simulink library "gasLibrary"  (R2019a)
settings: Solver=VariableStepAuto  StartTime=0.0  StopTime=10.0  RelTol=1e-3
values from neighbouring files (symbols this model uses):
  loadControlFlag = "on"    [gas_v1.m]
undefined symbols (not defined in the file or in its folder): f
libraries: fl_lib x34, nesl_utility x12, instrumentlib x5
settings Model: Creator=dzimm  LastModifiedBy=brandt

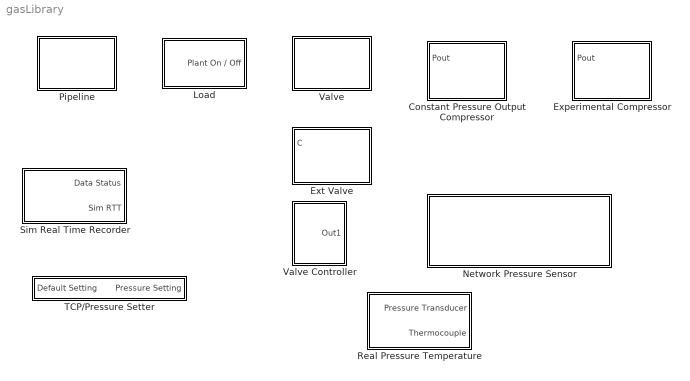
== system gasLibrary ==
  Constant Pressure Output Compressor : Subsystem  mask{xferNum=1, xferDen=[1800 1], delaySeconds=1, efficiency=0.3}
      mask prompts: xferNum "Plant Transfer Function Numerator (vector)"; xferDen "Plant Transfer Function Denominator (vector)"; delaySeconds "Response Delay (s)"; efficiency "Full Efficiency (-)"
  Experimental Compressor : Subsystem  AncestorBlock=gasLibrary/Constant Pressure Output Compressor  mask{xferNum=1, xferDen=[1800 1], delaySeconds=1, efficiency=0.3}
      mask prompts: xferNum "Plant Transfer Function Numerator (vector)"; xferDen "Plant Transfer Function Denominator (vector)"; delaySeconds "Response Delay (s)"; efficiency "Full Efficiency (-)"
  Ext Valve : Subsystem  AncestorBlock=gasLibrary/Valve  mask{valveRow=[], valveState="on"}
      mask prompts: valveRow "Valve Control (table row)"; valveState "Valve Simulation Control ('on' 'off' 'initial')"
      mask init:
      | if(isempty(valveRow)||isnumeric(valveRow))
      |     valveName="Valve";
      |     valveTime=[0 1e6]';
      |     valveSetting=[0 0]';
      |     D=20;           % size of the valve
      |     Dmax=D-1;       % maximum port opening
      |     textColor='red';
      | else
      |     valveName=valveRow.Name;
      |     t=valveRow.Time{1};
      |     g=valveRow.State{1};
      |     D=valveRow.PortDiameter;
      |     Dmax=valveRow.MaxValveDiameter;
      |     switch(lower(valveState))
      |         case "on"
      |             valveTime=t(:);
      |             valveSetting=g(:);
      |             textColor='green';
      |         case "off"
      |             valveTime=[0 1e6]';
      |             valveSetting=[1 1]';
      |             textColor='red';
      |         case "initial"
      |             valveTime=[0 1e6 ]';   % ramp gas on over one day
      |             valveSetting=[g(1)    g(1)]';     % gas ends at initial value
      |             textColor='blue';
      |         otherwise
      |             fprintf("Cannot initialize\n");
      |             textColor='green';
      |     end
      | end
      mask Display:
      | set_param(gcb,'Name',valveName);
      | color(textColor);
      | if(valveState=="off")
      |     vLabel="bypass";
      | else
      |     vLabel="active";
      | end
      | text(0.1,0.8,sprintf("%s (%1d in)",vLabel,D))
      | plot([0.2 0.9],[0.3 0.3]);
      | plot([0.2 0.2],[0.1 0.6]);
      | plot(valveTime/max(valveTime)*0.65+0.2,double(valveSetting)*0.4+0.15);
  Load : Subsystem  mask{loadRow=0, loadState=loadControlFlag}
      mask prompts: loadRow "Load Parameters (table row)"; loadState "Load Simulation Control ('on','off','initial')"
      mask init:
      | if(isempty(loadRow)||isnumeric(loadRow))
      |     loadName="Load";
      |     gasTime=[0 1e6]';
      |     gasLoad=[0 0]';
      |     textColor='red';
      |     pNominal=300;
      |     pCutoff=150;
      | else
      |     loadName=loadRow.Name;
      |     t=loadRow.Time{1};
      |     g=loadRow.Load{1};
      |     pNominal=loadRow.NominalPressure;
      |     pCutoff=loadRow.PressureCutoff;
      |     switch(lower(loadState))
      |         case "on"
      |             gasTime=t(:);
      |             gasLoad=g(:);
      |             textColor='green';
      |         case "off"
      |             gasTime=[0 1e6]';
      |             gasLoad=[0 0]';
      |             textColor='red';
      |         case "initial"
      |             gasTime=[0 24*3600 1e6 ]';   % ramp gas on over one day
      |             gasLoad=[0 g(1)    g(1)]';     % gas ends at initial value
      |             textColor='blue';
      |         otherwise
      |             fprintf("Cannot initialize\n");
      |             textColor='green';
      |     end
      | end
      mask Display:
      | tMax=max([gasTime(end)]);
      | set_param(gcb,'Name',loadName);
      | color(textColor);
      | text(0.1,0.8,sprintf("%s / %2.1f kg/s",loadState,max(gasLoad)))
      | plot([0.2 0.8],[0.1 0.1]);
      | plot([0.2 0.2],[0.1 0.6]);
      | plot(gasTime/tMax*0.6+0.2,gasLoad/max(gasLoad)*0.5+0.1);
  "Network Pressure Sensor " : Subsystem
  Pipeline : Subsystem  mask{pipeRow=[]}
      mask prompts: pipeRow "Pipeilne Configuration (table row)"
      mask init:
      | if(isempty(pipeRow))
      |     pipeName="Pipeline";
      |     D=24;
      |     L=50;
      |     Pstart=300;
      | else
      |     pipeName=pipeRow.Name;
      |     D=pipeRow.DiameterInch;
      |     L=pipeRow.LengthMiles;
      |     Pstart=pipeRow.StartPressurePSI;
      | end
      mask Display:
      | fprintf('%1d"\n%1d miles\n%1d psi',D,L,Pstart)
      | set_param(gcb,'Name',pipeName)
  Real Pressure Temperature : Subsystem  AncestorBlock=gasLibrary/Physical to Real Pressure Temperature
  Sim Real Time Recorder : Subsystem
  TCP/Pressure Setter : Subsystem
  Valve : Subsystem  mask{valveRow=[], valveState="on"}
      mask prompts: valveRow "Valve Control (table row)"; valveState "Valve Simulation Control ('on' 'off' 'initial')"
      mask init: same as gasLibrary/Ext Valve
      mask Display:
      | set_param(gcb,'Name',valveName);
      | color(textColor);
      | if(valveState=="off")
      |     vLabel="bypass";
      | else
      |     vLabel="active";
      | end
      | text(0.1,0.8,sprintf("%s (%1d in)",vLabel,D))
      | plot([0.2 0.9],[0.3 0.3]);
      | plot([0.2 0.2],[0.1 0.6]);
      | plot(valveTime/max(valveTime)*0.65+0.2,double(valveSetting)*0.4+0.15);
  Valve Controller : Subsystem

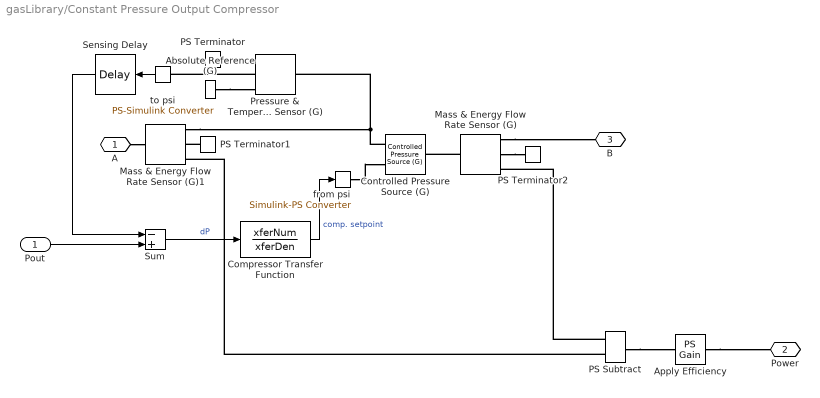
== system gasLibrary/Constant Pressure Output Compressor ==
  Pout : Inport
  Absolute Reference (G) : fl_lib/Gas/Elements/Absolute Reference (G)
      settings: SourceProductName=Simscape  SourceProductBaseCode=SS
  Apply Efficiency : fl_lib/Physical Signals/Functions/PS Gain  gain=1/efficiency
  Compressor Transfer Function : TransferFcn  Numerator=xferNum  Denominator=xferDen
  Controlled Pressure Source (G) : fl_lib/Gas/Sources/Controlled Pressure Source (G)  power_spec=1  area_A=24^2*pi/4 in^2  area_B=24^2*pi/4 in^2  mdot_A_specify=off  mdot_A_priority=None  mdot_A=1e-6 kg/s  mdot_A_nominal_specify=off  mdot_A_nominal_unit=kg/s  mdot_A_nominal_value=1
      settings: SourceProductName=Simscape  SourceProductBaseCode=SS
  Mass & Energy Flow Rate Sensor (G) : fl_lib/Gas/Sensors/Mass & Energy Flow Rate Sensor (G)
      settings: SourceProductName=Simscape  SourceProductBaseCode=SS
  Mass & Energy Flow Rate Sensor (G)1 : fl_lib/Gas/Sensors/Mass & Energy Flow Rate Sensor (G)
      settings: SourceProductName=Simscape  SourceProductBaseCode=SS
  PS Subtract : fl_lib/Physical Signals/Functions/PS Subtract
      settings: SourceProductName=Simscape
  PS Terminator : fl_lib/Physical Signals/Sinks/PS Terminator
      settings: SourceProductName=Simscape
  PS Terminator1 : fl_lib/Physical Signals/Sinks/PS Terminator
      settings: SourceProductName=Simscape
  PS Terminator2 : fl_lib/Physical Signals/Sinks/PS Terminator
      settings: SourceProductName=Simscape
  Pressure & Temperature Sensor (G) : fl_lib/Gas/Sensors/Pressure & Temperature Sensor (G)
      settings: SourceProductName=Simscape  SourceProductBaseCode=SS
  Sensing Delay : TransportDelay  DelayTime=delaySeconds  TransDelayFeedthrough=on
  Sum : Sum  Inputs=-+
  from psi : nesl_utility/Simulink-PS Converter  PhysicalDomain=network_engine_domain  SubClassName=ps_input  LeftPortType=input  RightPortType=output  PseudoPeriodic=off  Frequencies=[]  NoiseDistribution=none  NoiseParameters=[]  Unit=psi  AffineConversion=off  FilteringAndDerivatives=provide  SimscapeFilterOrder=1  InputFilterTimeConstant=0.001  UdotUserProvided=0
  to psi : nesl_utility/PS-Simulink Converter  PhysicalDomain=network_engine_domain  SubClassName=ps_output  LeftPortType=input  RightPortType=output  PseudoPeriodic=off  Frequencies=[]  Unit=psi  AffineConversion=off
  A : PMIOPort  Side=Left
  Power : PMIOPort  Port=2  Side=Right
  B : PMIOPort  Port=3  Side=Right
  wires:
  Pout/1 -> Sum/2
  Sum/1 -> Compressor Transfer Function/1  "dP"
  Compressor Transfer Function/1 -> from psi/1  "comp. setpoint"
  Sensing Delay/1 -> Sum/1
  to psi/1 -> Sensing Delay/1
  connections:
  Absolute Reference (G)/LConn1 -- Pressure & Temperature Sensor (G)/RConn1
  Pressure & Temperature Sensor (G)/RConn2 -- to psi/LConn1
  from psi/RConn1 -- Controlled Pressure Source (G)/LConn2
  PS Terminator/LConn1 -- Pressure & Temperature Sensor (G)/RConn3
  Controlled Pressure Source (G)/LConn1 -- Mass & Energy Flow Rate Sensor (G)1/RConn1 -- Pressure & Temperature Sensor (G)/LConn1
  Mass & Energy Flow Rate Sensor (G)/LConn1 -- Controlled Pressure Source (G)/RConn1
  Mass & Energy Flow Rate Sensor (G)/RConn1 -- B/RConn1
  A/RConn1 -- Mass & Energy Flow Rate Sensor (G)1/LConn1
  PS Terminator1/LConn1 -- Mass & Energy Flow Rate Sensor (G)1/RConn2
  Mass & Energy Flow Rate Sensor (G)/RConn2 -- PS Terminator2/LConn1
  PS Subtract/LConn1 -- Mass & Energy Flow Rate Sensor (G)/RConn3
  PS Subtract/LConn2 -- Mass & Energy Flow Rate Sensor (G)1/RConn3
  PS Subtract/RConn1 -- Apply Efficiency/LConn1
  Apply Efficiency/RConn1 -- Power/RConn1

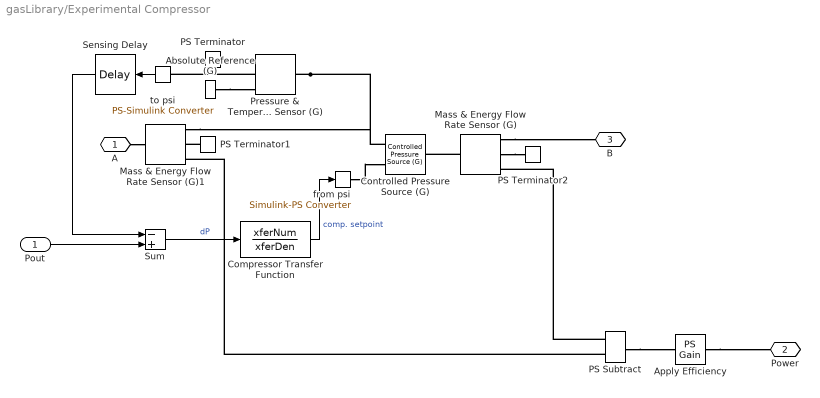
== system gasLibrary/Experimental Compressor ==
  Pout : Inport
  Absolute Reference (G) : fl_lib/Gas/Elements/Absolute Reference (G)
      settings: SourceProductName=Simscape  SourceProductBaseCode=SS
  Apply Efficiency : fl_lib/Physical Signals/Functions/PS Gain  gain=1/efficiency
  Compressor Transfer Function : TransferFcn  Numerator=xferNum  Denominator=xferDen
  Controlled Pressure Source (G) : fl_lib/Gas/Sources/Controlled Pressure Source (G)  power_spec=1  area_A=24^2*pi/4 in^2  area_B=24^2*pi/4 in^2  mdot_A_specify=off  mdot_A_priority=None  mdot_A=1e-6 kg/s  mdot_A_nominal_specify=off  mdot_A_nominal_unit=kg/s  mdot_A_nominal_value=1
      settings: SourceProductName=Simscape  SourceProductBaseCode=SS
  Mass & Energy Flow Rate Sensor (G) : fl_lib/Gas/Sensors/Mass & Energy Flow Rate Sensor (G)
      settings: SourceProductName=Simscape  SourceProductBaseCode=SS
  Mass & Energy Flow Rate Sensor (G)1 : fl_lib/Gas/Sensors/Mass & Energy Flow Rate Sensor (G)
      settings: SourceProductName=Simscape  SourceProductBaseCode=SS
  PS Subtract : fl_lib/Physical Signals/Functions/PS Subtract
      settings: SourceProductName=Simscape
  PS Terminator : fl_lib/Physical Signals/Sinks/PS Terminator
      settings: SourceProductName=Simscape
  PS Terminator1 : fl_lib/Physical Signals/Sinks/PS Terminator
      settings: SourceProductName=Simscape
  PS Terminator2 : fl_lib/Physical Signals/Sinks/PS Terminator
      settings: SourceProductName=Simscape
  Pressure & Temperature Sensor (G) : fl_lib/Gas/Sensors/Pressure & Temperature Sensor (G)
      settings: SourceProductName=Simscape  SourceProductBaseCode=SS
  Sensing Delay : TransportDelay  DelayTime=delaySeconds  TransDelayFeedthrough=on
  Sum : Sum  Inputs=-+
  from psi : nesl_utility/Simulink-PS Converter  PhysicalDomain=network_engine_domain  SubClassName=ps_input  LeftPortType=input  RightPortType=output  PseudoPeriodic=off  Frequencies=[]  NoiseDistribution=none  NoiseParameters=[]  Unit=psi  AffineConversion=off  FilteringAndDerivatives=provide  SimscapeFilterOrder=1  InputFilterTimeConstant=0.001  UdotUserProvided=0
  to psi : nesl_utility/PS-Simulink Converter  PhysicalDomain=network_engine_domain  SubClassName=ps_output  LeftPortType=input  RightPortType=output  PseudoPeriodic=off  Frequencies=[]  Unit=psi  AffineConversion=off
  A : PMIOPort  Side=Left
  Power : PMIOPort  Port=2  Side=Right
  B : PMIOPort  Port=3  Side=Right
  wires:
  to psi/1 -> Sensing Delay/1
  Sensing Delay/1 -> Sum/1
  Compressor Transfer Function/1 -> from psi/1  "comp. setpoint"
  Sum/1 -> Compressor Transfer Function/1  "dP"
  Pout/1 -> Sum/2
  connections:
  Apply Efficiency/RConn1 -- Power/RConn1
  PS Subtract/RConn1 -- Apply Efficiency/LConn1
  PS Subtract/LConn2 -- Mass & Energy Flow Rate Sensor (G)1/RConn3
  PS Subtract/LConn1 -- Mass & Energy Flow Rate Sensor (G)/RConn3
  Mass & Energy Flow Rate Sensor (G)/RConn2 -- PS Terminator2/LConn1
  PS Terminator1/LConn1 -- Mass & Energy Flow Rate Sensor (G)1/RConn2
  A/RConn1 -- Mass & Energy Flow Rate Sensor (G)1/LConn1
  Mass & Energy Flow Rate Sensor (G)/RConn1 -- B/RConn1
  Mass & Energy Flow Rate Sensor (G)/LConn1 -- Controlled Pressure Source (G)/RConn1
  Pressure & Temperature Sensor (G)/LConn1 -- Mass & Energy Flow Rate Sensor (G)1/RConn1 -- Controlled Pressure Source (G)/LConn1
  PS Terminator/LConn1 -- Pressure & Temperature Sensor (G)/RConn3
  from psi/RConn1 -- Controlled Pressure Source (G)/LConn2
  Pressure & Temperature Sensor (G)/RConn2 -- to psi/LConn1
  Absolute Reference (G)/LConn1 -- Pressure & Temperature Sensor (G)/RConn1

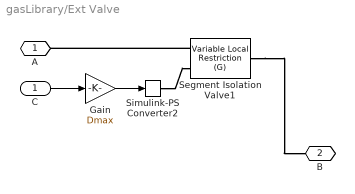
== system gasLibrary/Ext Valve ==
  C : Inport
  Gain : Gain  Gain=Dmax
  Segment Isolation Valve1 : fl_lib/Gas/Elements/Variable Local Restriction (G)  min_area=1e-4 in^2  max_area=pi*(Dmax-1)^2/4 in^2  area=pi*D^2/4 in^2  Cd=0.64  B_lam=0.999  mdot_A_specify=off  mdot_A_priority=None  mdot_A=1e-6 kg/s  mdot_A_nominal_specify=off  mdot_A_nominal_unit=kg/s  mdot_A_nominal_value=1
      settings: SourceProductName=Simscape  SourceProductBaseCode=SS
  Simulink-PS Converter2 : nesl_utility/Simulink-PS Converter  PhysicalDomain=network_engine_domain  SubClassName=ps_input  LeftPortType=input  RightPortType=output  PseudoPeriodic=off  Frequencies=[]  NoiseDistribution=none  NoiseParameters=[]  Unit=in^2  AffineConversion=off  FilteringAndDerivatives=provide  SimscapeFilterOrder=1  InputFilterTimeConstant=0.001  UdotUserProvided=0
  A : PMIOPort  Side=Left
  B : PMIOPort  Port=2  Side=Right
  wires:
  C/1 -> Gain/1
  Gain/1 -> Simulink-PS Converter2/1
  connections:
  Segment Isolation Valve1/RConn1 -- B/RConn1
  Segment Isolation Valve1/LConn1 -- A/RConn1
  Simulink-PS Converter2/RConn1 -- Segment Isolation Valve1/LConn2

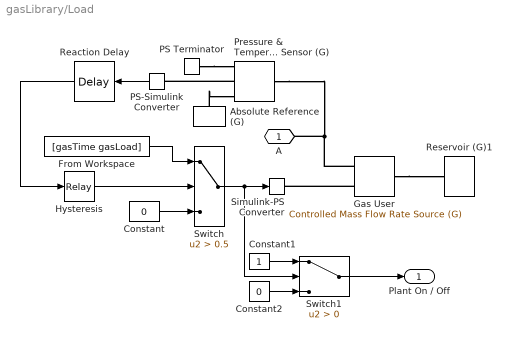
== system gasLibrary/Load ==
  Absolute Reference (G) : fl_lib/Gas/Elements/Absolute Reference (G)
      settings: SourceProductName=Simscape  SourceProductBaseCode=SS
  Constant : Constant  Value=0
  Constant1 : Constant
  Constant2 : Constant  Value=0
  From Workspace : FromWorkspace  VariableName=[gasTime gasLoad]  SampleTime=0  OutputAfterFinalValue=Holding final value
  Gas User : fl_lib/Gas/Sources/Controlled Mass Flow Rate Source (G)  power_spec=1  area_A=24^2*pi/4 in^2  area_B=20^2*pi/4 in^2  mdot_A_specify=on  mdot_A_priority=None  mdot_A=20 kg/s  mdot_A_nominal_specify=off  mdot_A_nominal_unit=kg/s  mdot_A_nominal_value=1
      settings: SourceProductName=Simscape  SourceProductBaseCode=SS
  Hysteresis : Relay  OnSwitchValue=pCutoff*1.05  OffSwitchValue=pCutoff
  PS Terminator : fl_lib/Physical Signals/Sinks/PS Terminator
      settings: SourceProductName=Simscape
  PS-Simulink Converter : nesl_utility/PS-Simulink Converter  PhysicalDomain=network_engine_domain  SubClassName=ps_output  LeftPortType=input  RightPortType=output  PseudoPeriodic=off  Frequencies=[]  Unit=psi  AffineConversion=off
  Pressure & Temperature Sensor (G) : fl_lib/Gas/Sensors/Pressure & Temperature Sensor (G)
      settings: SourceProductName=Simscape  SourceProductBaseCode=SS
  Reaction Delay : TransportDelay  DelayTime=60  InitialOutput=pNominal
  Reservoir (G)1 : fl_lib/Gas/Elements/Reservoir (G)  pressure_spec=2  reservoir_pressure=300 psi  reservoir_temperature=25 degC  area_A=pi*25^2/4 in^2
      settings: SourceProductName=Foundation Library
  Simulink-PS Converter : nesl_utility/Simulink-PS Converter  PhysicalDomain=network_engine_domain  SubClassName=ps_input  LeftPortType=input  RightPortType=output  PseudoPeriodic=off  Frequencies=[]  NoiseDistribution=none  NoiseParameters=[]  Unit=1  AffineConversion=off  FilteringAndDerivatives=provide  SimscapeFilterOrder=1  InputFilterTimeConstant=0.001  UdotUserProvided=0
  Switch : Switch  Criteria=u2 > Threshold  Threshold=0.5
  Switch1 : Switch  Criteria=u2 > Threshold
  A : PMIOPort  Side=Left
  Plant On / Off : Outport
  wires:
  Reaction Delay/1 -> Hysteresis/1
  PS-Simulink Converter/1 -> Reaction Delay/1
  From Workspace/1 -> Switch/1
  Constant/1 -> Switch/3
  Hysteresis/1 -> Switch/2
  Switch/1 -> Switch1/2, Simulink-PS Converter/1
  Constant2/1 -> Switch1/3
  Switch1/1 -> Plant On / Off/1
  Constant1/1 -> Switch1/1
  connections:
  Gas User/RConn1 -- Reservoir (G)1/LConn1
  Gas User/LConn1 -- Pressure & Temperature Sensor (G)/LConn1 -- A/RConn1
  Gas User/LConn2 -- Simulink-PS Converter/RConn1
  PS Terminator/LConn1 -- Pressure & Temperature Sensor (G)/RConn3
  Absolute Reference (G)/LConn1 -- Pressure & Temperature Sensor (G)/RConn1
  Pressure & Temperature Sensor (G)/RConn2 -- PS-Simulink Converter/LConn1

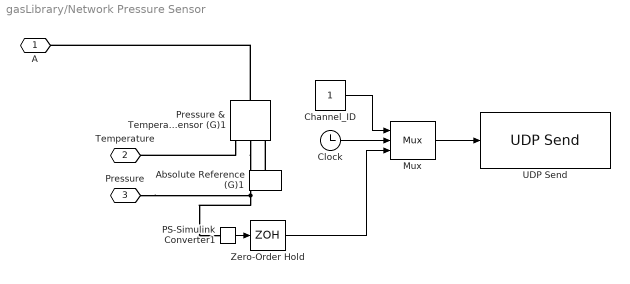
== system gasLibrary/Network Pressure Sensor  ==
  Absolute Reference (G)1 : fl_lib/Gas/Elements/Absolute Reference (G)
      settings: SourceProductName=Simscape  SourceProductBaseCode=SS
  Channel_ID : Constant
  Clock : Clock
  Mux : Mux  Inputs=3
      settings: DisplayOption=signals
  PS-Simulink Converter1 : nesl_utility/PS-Simulink Converter  PhysicalDomain=network_engine_domain  SubClassName=ps_output  LeftPortType=input  RightPortType=output  PseudoPeriodic=off  Frequencies=[]  Unit=1  AffineConversion=off
  Pressure & Temperature Sensor (G)1 : fl_lib/Gas/Sensors/Pressure & Temperature Sensor (G)
      settings: SourceProductName=Simscape  SourceProductBaseCode=SS
  UDP Send : instrumentlib/UDP Send  Host=localhost  Port=7070  LocalPort=-1  EnablePortSharing=off  ByteOrder=BigEndian  OutputDatagramPacketSize=512  EnableBlockingMode=on  LocalAddress=0.0.0.0
      settings: SourceProductName=Instrument Control Toolbox
  Zero-Order Hold : ZeroOrderHold  SampleTime=300
  A : PMIOPort  Side=Left
  Temperature : PMIOPort  Port=2  Side=Right
  Pressure : PMIOPort  Port=3  Side=Right
  wires:
  PS-Simulink Converter1/1 -> Zero-Order Hold/1
  Zero-Order Hold/1 -> Mux/3
  Mux/1 -> UDP Send/1
  Clock/1 -> Mux/2
  Channel_ID/1 -> Mux/1
  connections:
  Absolute Reference (G)1/LConn1 -- Pressure & Temperature Sensor (G)1/RConn1
  Pressure & Temperature Sensor (G)1/RConn2 -- PS-Simulink Converter1/LConn1 -- Pressure/RConn1
  Pressure & Temperature Sensor (G)1/LConn1 -- A/RConn1
  Pressure & Temperature Sensor (G)1/RConn3 -- Temperature/RConn1

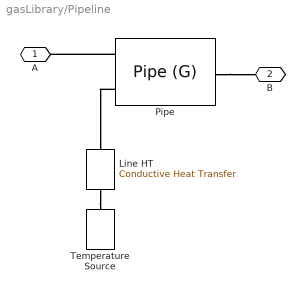
== system gasLibrary/Pipeline ==
  Line HT : fl_lib/Thermal/Thermal Elements/Conductive Heat Transfer  area=pi*(D/12)*(L*5280) ft^2  thickness=0.35 in  th_cond=54 W/(m*K)  T_specify=off  T_priority=None  T=0 K  T_nominal_specify=off  T_nominal_unit=K  T_nominal_value=1  Q_specify=off  Q_priority=None  Q=0 W  Q_nominal_specify=off  Q_nominal_unit=W  Q_nominal_value=1
      settings: SourceProductName=Simscape
  Pipe : fl_lib/Gas/Elements/Pipe (G)  length=L mi  area=D^2*pi/4 in^2  Dh=D in  length_add=100 ft  roughness=0.0018 in  Re_lam=2000  Re_tur=4000  shape_factor=64  Nu_lam=3.66  p_pipe_specify=on  p_pipe_priority=High  p_pipe=Pstart psi  p_pipe_nominal_specify=off  p_pipe_nominal_unit=MPa  p_pipe_nominal_value=1  T_pipe_specify=on  T_pipe_priority=High  T_pipe=25 degC  T_pipe_nominal_specify=off  T_pipe_nominal_unit=K  T_pipe_nominal_value=1  rho_pipe_specify=off  rho_pipe_priority=None  rho_pipe=14.4 kg/m^3  rho_pipe_nominal_specify=off  rho_pipe_nominal_unit=kg/m^3  rho_pipe_nominal_value=1
      settings: SourceProductName=Simscape  SourceProductBaseCode=SS
  Temperature Source : fl_lib/Thermal/Thermal Sources/Temperature Source  temperature=25 degC
      settings: SourceProductName=Simscape
  A : PMIOPort  Side=Left
  B : PMIOPort  Port=2  Side=Right
  connections:
  Pipe/RConn1 -- B/RConn1
  Pipe/LConn2 -- Line HT/RConn1
  Line HT/LConn1 -- Temperature Source/LConn1
  Pipe/LConn1 -- A/RConn1

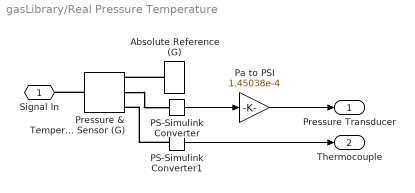
== system gasLibrary/Real Pressure Temperature ==
  Absolute Reference (G) : fl_lib/Gas/Elements/Absolute Reference (G)
      settings: SourceProductName=Simscape  SourceProductBaseCode=SS
  PS-Simulink Converter : nesl_utility/PS-Simulink Converter  PhysicalDomain=network_engine_domain  SubClassName=ps_output  LeftPortType=input  RightPortType=output  PseudoPeriodic=off  Frequencies=[]  Unit=1  AffineConversion=off
  PS-Simulink Converter1 : nesl_utility/PS-Simulink Converter  PhysicalDomain=network_engine_domain  SubClassName=ps_output  LeftPortType=input  RightPortType=output  PseudoPeriodic=off  Frequencies=[]  Unit=1  AffineConversion=off
  Pa to PSI : Gain  Gain=1.45038e-4
  Pressure & Temperature Sensor (G) : fl_lib/Gas/Sensors/Pressure & Temperature Sensor (G)
      settings: SourceProductName=Simscape  SourceProductBaseCode=SS
  Signal In : PMIOPort  Side=Left
  Pressure Transducer : Outport
  Thermocouple : Outport  Port=2
  wires:
  PS-Simulink Converter/1 -> Pa to PSI/1
  PS-Simulink Converter1/1 -> Thermocouple/1
  Pa to PSI/1 -> Pressure Transducer/1
  connections:
  Pressure & Temperature Sensor (G)/LConn1 -- Signal In/RConn1
  Absolute Reference (G)/LConn1 -- Pressure & Temperature Sensor (G)/RConn1
  PS-Simulink Converter1/LConn1 -- Pressure & Temperature Sensor (G)/RConn3
  Pressure & Temperature Sensor (G)/RConn2 -- PS-Simulink Converter/LConn1

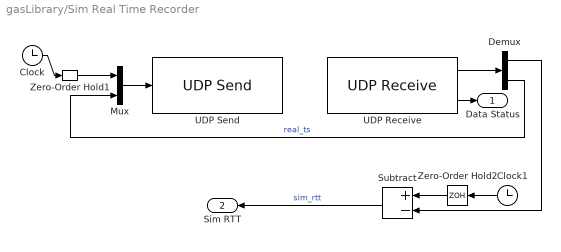
== system gasLibrary/Sim Real Time Recorder ==
  Clock : Clock
  Clock1 : Clock
  Demux : Demux  Outputs=2
  Mux : Mux  Inputs=2
  Subtract : Sum  Inputs=+-
  UDP Receive : instrumentlib/UDP Receive  Priority=2  Host=localhost  Port=8080  LocalPort=8081  EnablePortSharing=off  GetLatestData=off  DataSize="[2  1]"  DataType=double  ASCIIFormatting=%f,  Terminator=LF  ByteOrder=BigEndian  EnableBlockingMode=off  Timeout=50  SampleTime=0.01  LocalAddress=localhost
      settings: SourceProductName=Instrument Control Toolbox
  UDP Send : instrumentlib/UDP Send  Priority=1  Host=localhost  Port=8080  LocalPort=-1  EnablePortSharing=off  ByteOrder=BigEndian  OutputDatagramPacketSize=24  EnableBlockingMode=on  LocalAddress=0.0.0.0
      settings: SourceProductName=Instrument Control Toolbox
  Zero-Order Hold1 : ZeroOrderHold  SampleTime=-1
  Zero-Order Hold2 : ZeroOrderHold  SampleTime=-1
  Data Status : Outport
  Sim RTT : Outport  Port=2
  wires:
  Subtract/1 -> Sim RTT/1  "sim_rtt"
  Zero-Order Hold1/1 -> Mux/1
  Zero-Order Hold2/1 -> Subtract/1
  Mux/1 -> UDP Send/1
  UDP Receive/2 -> Data Status/1
  Demux/2 -> Mux/2  "real_ts"
  UDP Receive/1 -> Demux/1
  Demux/1 -> Subtract/2
  Clock/1 -> Zero-Order Hold1/1
  Clock1/1 -> Zero-Order Hold2/1

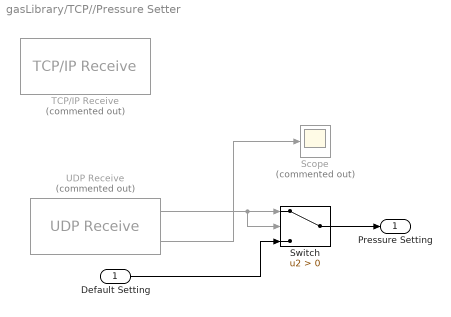
== system gasLibrary/TCP//Pressure Setter ==
  Default Setting : Inport
  Scope : Scope  Commented=on
  Switch : Switch  Criteria=u2 > Threshold
  TCP/IP Receive : instrumentlib/TCP//IP Receive  Commented=on  Host=localhost  Port=7777  DataSize=[1 1]  EnableBlockingMode=off  Timeout=10  SampleTime=300  DataType=int16  ByteOrder=BigEndian  ASCIIFormatting=%f,  Terminator=LF
      settings: SourceProductName=Instrument Control Toolbox
  UDP Receive : instrumentlib/UDP Receive  Commented=on  Host=localhost  Port=9090  LocalPort=7777  EnablePortSharing=off  GetLatestData=on  DataSize=[1 1]  DataType=int16  ASCIIFormatting=%f,  Terminator=LF  ByteOrder=BigEndian  EnableBlockingMode=off  Timeout=10  SampleTime=300  LocalAddress=localhost
      settings: SourceProductName=Instrument Control Toolbox
  "Pressure Setting " : Outport
  wires:
  Default Setting/1 -> Switch/3
  Switch/1 -> "Pressure Setting "/1
  UDP Receive/1 -> Switch/2, Switch/1
  UDP Receive/2 -> Scope/1

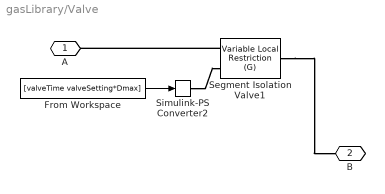
== system gasLibrary/Valve ==
  From Workspace : FromWorkspace  VariableName=[valveTime valveSetting*Dmax]  SampleTime=0  OutputAfterFinalValue=Holding final value
  Segment Isolation Valve1 : fl_lib/Gas/Elements/Variable Local Restriction (G)  min_area=1e-4 in^2  max_area=pi*(Dmax-1)^2/4 in^2  area=pi*D^2/4 in^2  Cd=0.64  B_lam=0.999  mdot_A_specify=off  mdot_A_priority=None  mdot_A=1e-6 kg/s  mdot_A_nominal_specify=off  mdot_A_nominal_unit=kg/s  mdot_A_nominal_value=1
      settings: SourceProductName=Simscape  SourceProductBaseCode=SS
  Simulink-PS Converter2 : nesl_utility/Simulink-PS Converter  PhysicalDomain=network_engine_domain  SubClassName=ps_input  LeftPortType=input  RightPortType=output  PseudoPeriodic=off  Frequencies=[]  NoiseDistribution=none  NoiseParameters=[]  Unit=in^2  AffineConversion=off  FilteringAndDerivatives=provide  SimscapeFilterOrder=1  InputFilterTimeConstant=0.001  UdotUserProvided=0
  A : PMIOPort  Side=Left
  B : PMIOPort  Port=2  Side=Right
  wires:
  From Workspace/1 -> Simulink-PS Converter2/1
  connections:
  Segment Isolation Valve1/RConn1 -- B/RConn1
  Segment Isolation Valve1/LConn1 -- A/RConn1
  Simulink-PS Converter2/RConn1 -- Segment Isolation Valve1/LConn2

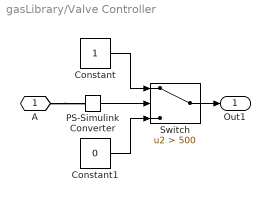
== system gasLibrary/Valve Controller ==
  Constant : Constant
  Constant1 : Constant  Value=0
  PS-Simulink Converter : nesl_utility/PS-Simulink Converter  PhysicalDomain=network_engine_domain  SubClassName=ps_output  LeftPortType=input  RightPortType=output  PseudoPeriodic=off  Frequencies=[]  Unit=1  AffineConversion=off
  Switch : Switch  Criteria=u2 > Threshold  Threshold=500
  A : PMIOPort  Side=Left
  Out1 : Outport
  wires:
  Constant1/1 -> Switch/3
  Switch/1 -> Out1/1
  Constant/1 -> Switch/1
  PS-Simulink Converter/1 -> Switch/2
  connections:
  A/RConn1 -- PS-Simulink Converter/LConn1
